simulink model "PubIfDecisionTOS_MDL"  (R2020b)
settings: configuration reference "DspaceConfig" (kept outside this file)
PostLoadFcn:
  | if any(exist('dsrtsu_mdlpostloadfcn', 'file') ~= 0), dsrtsu_mdlpostloadfcn('Execute', bdroot); end
InitFcn:
  | , if any(exist('dsmpb_private', 'file') ~= 0), dsmpb_private('dsmpb_mdlclblib', 'Init', bdroot); end,
undefined symbols (not defined in the file or in its folder): C_TOS_ACCEgoRAxletoFbumplength_m, C_TOS_ACCTargetFront_Flag, C_TOS_AEBJAPedObjDxThre_Val, C_TOS_AEBJAPedObjDyThre_Val, C_TOS_AEBJATargetSize_Val, C_TOS_AEBJAVehObjDxThre_Val, C_TOS_AEBJAVehObjDyThre_Val, C_TOS_AEBJuncPedTargetSize_Val, C_TOS_AEBLatObjDxThre_Val, C_TOS_AEBLatPedDyThre_Val, C_TOS_AEBLatTargetSize_Val, C_TOS_AEBLongTargetInEgoFront_Flag, C_TOS_axAbsGround_Parameter, C_TOS_CameraConfirmedFlag, C_TOS_CNsubjWidth, C_TOS_CurrentLaneCoreMinWidth_Val, C_TOS_CutInProb_Val_Zero, C_TOS_CutOutProb_Val_Zero, C_TOS_D2R_Val, C_TOS_DefaultValueObjectToCenterLine_dy, C_TOS_EgoCarWidth_Val, C_TOS_EgoDxRefPoint_m, C_TOS_EgoRAxletoFbumplength_m, C_TOS_HalfWidthVehicle_Con, C_TOS_HWA_CurrentLaneFlag, C_TOS_HWA_LeftLaneFlag, C_TOS_HWA_MovingDir_Vaild, C_TOS_HWA_MovState_Vaild, C_TOS_HWA_RightLaneFlag, C_TOS_LaneLineCourseErrorFront, C_TOS_LaneLineCourseErrorRear, C_TOS_MotorbikeDefaultWidth_m, C_TOS_NumberOfEffectiveTargets, C_TOS_Obj_Age_Val, C_TOS_Objdx_Constraint_Val, C_TOS_ObjectDefaultWidth_m, C_TOS_ObjInCurrentLane_Val, C_TOS_ObjInCurrentLaneValid, C_TOS_ObjInLeftLaneValid, C_TOS_ObjInRightLaneValid, C_TOS_ObjNotInCurrentLane_Val, C_TOS_ObjNotREElementType, C_TOS_ObjPredictDis_dy_ConstantVal_Zeros, C_TOS_ObjToCenterLine_ConstantVal_Zeros, C_TOS_OFMObjIDInvilad_Val, C_TOS_PIL_LatDisCons_Val_zero, C_TOS_PIL_ObjectCutInFlag_b, C_TOS_PIL_ObjectCutOutFlag_b, C_TOS_PIL_ObjLaneProb_al_Val, C_TOS_PP_ObjFusType_FC_Confirm_b, C_TOS_PP_ObjFusType_FC_FR_Confirm_b, C_TOS_PP_ObjFusType_FR_Confirm_b, C_TOS_RE_80BoolDefault_Val, C_TOS_RE_80Single181Default_Val, C_TOS_RE_80Single255Default_Val, C_TOS_RE_80Uint8Default_Val, C_TOS_RE_D2R, C_TOS_RE_D_180_Val, C_TOS_RE_InvalidObjectID_Val, C_TOS_RE_InvalidTargetChainDir_Val ... (+142)
libraries: simulink x1650, TOS_LIB x361, canfdmsglib x14
(part 7 of 69)

== system PubIfDecisionTOS_MDL/TOS_20201112/TOS_2012080320/TOS/ACC/TOS_ACCCurrentLane ==
  TOSAAt_OFM_TIL_VIE : Inport
  ACCTargetInfor : Subsystem
  ACC_CurrentLane_Target : Subsystem
  ACC_Object_PreConfirm : Subsystem
  Bus Selector : BusSelector  OutputSignals=IDP0,dxP0
  Bus Selector1 : BusSelector  OutputSignals=VIE_SignalVerification.vxvRefMs,OFM_SignalVerification,TOS_AddAttributes,TLJ_TargetInLaneValidityJudg.TOS_TLJ_SameLaneConfirm_Flag,TOS_ProbInLaneCalculat,TOS_VCAN_SignalVerification,LM_SignalVerification.TOS_LM_LR_Bus.LM_LR_Line04.dDisStart,LM_SignalVerification.TOS_LM_LR_Bus.LM_LR_Line04.dDisEnd,LM_SignalVerification.TOS_LM_LR_Bus.LM_LR_Line05.dDisStart,LM_SignalVerification.TOS_LM_LR_Bus.LM_LR_Line05.dDisEnd,LM_SignalVerification.TOS_LM_LR_Bus.LM_LR_Line06.dDisStart,LM_SignalVerification.TOS_LM_LR_Bus.LM_LR_Line06.dDisEnd,LM_SignalVerification.TOS_LM_LR_Bus.LM_LR_Line04.pC2,LM_SignalVerification.TOS_LM_LR_Bus.LM_LR_Line05.pC2,LM_SignalVerification.TOS_LM_LR_Bus.LM_LR_Line06.pC2,LM_SignalVerification.TOS_LM_LR_Bus.LM_LR_Line04.fCamValid,LM_SignalVerification.TOS_LM_LR_Bus.LM_LR_Line05.fCamValid,LM_SignalVerification.TOS_LM_LR_Bus.LM_LR_Line06.fCamValid,LM_SignalVerification.TOS_LM_LR_Bus.LM_LR_Line04.pC0,LM_SignalVerification.TOS_LM_RL_Bus.LM_RL_Line04.pC0,LM_SignalVerification.TOS_LM_LR_Bus.LM_LR_Line04.pC1,LM_SignalVerification.TOS_LM_RL_Bus.LM_RL_Line04.pC1
  Bus Selector2 : BusSelector  OutputSignals=OFM_SignalVerification,TOS_AddAttributes,TOS_ProbInLaneCalculat
  Bus Selector3 : BusSelector  OutputSignals=IDP0,ObjMovingStateP0
  Bus Selector4 : BusSelector  OutputSignals=OFM_SignalVerification.Object_DX,OFM_SignalVerification.Object_ID
  Bus Selector5 : BusSelector  OutputSignals=TOS_AddAttributes.PP_ObjFusType_FC_FR_Confirm,TOS_AddAttributes.PP_ObjFusType_FR_Confirm,TOS_AddAttributes.PP_ObjFusType_FC_Confirm,OFM_SignalVerification.Object_ID,OFM_SignalVerification.Object_MovingState,OFM_SignalVerification.Object_DX,OFM_SignalVerification.Object_ObstacleProb,OFM_SignalVerification.Object_DY,OFM_SignalVerification.Object_Type,TLJ_TargetInLaneValidityJudg.TOS_TLJ_SameLaneConfirm_Flag,LM_SignalVerification.TOS_LM_LR_Bus.LM_LR_Line04.fCamValid,LM_SignalVerification.TOS_LM_LR_Bus.LM_LR_Line05.fCamValid,LM_SignalVerification.TOS_LM_LR_Bus.LM_LR_Line06.fCamValid,TOS_ProbInLaneCalculat.PIL_OverlapRatio,LM_SignalVerification.TOS_LM_LR_Bus.LM_LR_Line04.dDisStart,LM_SignalVerification.TOS_LM_LR_Bus.LM_LR_Line04.dDisEnd,LM_SignalVerification.TOS_LM_LR_Bus.LM_LR_Line05.dDisStart,LM_SignalVerification.TOS_LM_LR_Bus.LM_LR_Line05.dDisEnd,LM_SignalVerification.TOS_LM_LR_Bus.LM_LR_Line06.dDisStart,LM_SignalVerification.TOS_LM_LR_Bus.LM_LR_Line06.dDisEnd,PP_REElementType
  Bus Selector6 : BusSelector  OutputSignals=IDP1,ObjMovingStateP1
  Bus Selector7 : BusSelector  OutputSignals=TOS_ACC_P0_P1_TargetPre_SameLaneFlag,TOS_ACC_P0_P1_TargetPreFiltFlag
  Constant1 : Constant  Value=C_TOS_NumberOfEffectiveTargets  OutDataTypeStr=uint8
      settings: AttributesFormatString=C_TOS_NumberOfEffectiveTargets = 80
  MATLAB Function1 : MATLAB Function  TreatAsAtomicUnit=on
  Terminator1 : Terminator
  Terminator2 : Terminator
  Vector Concatenate : Concatenate
  TOS_ACCP0 : Outport  PortDimensions=1  BusOutputAsStruct=on
  TOS_ACCP1 : Outport  Port=2
  wires:
  ACCTargetInfor/2(TOS_ACCP1) -> TOS_ACCP1/1, [TOS_ACCP1]
  Bus Selector2/2 -> ACCTargetInfor/2(TOS_AddAttributes)  "<TOS_AddAttributes>"
  Bus Selector2/1 -> ACCTargetInfor/1(OFM_SignalVerification)  "<OFM_SignalVerification>"
  Bus Selector2/3 -> ACCTargetInfor/3(TOS_ProbInLaneCalculat)  "<TOS_ProbInLaneCalculat>"
  Bus Selector1/1 -> ACC_CurrentLane_Target/1(VIE_EgoVelocity)  "<vxvRefMs>"
  Bus Selector1/2 -> ACC_CurrentLane_Target/2(OFM_SignalVerification)  "<OFM_SignalVerification>"
  Bus Selector1/3 -> ACC_CurrentLane_Target/3(TOS_AddAttributes)  "<TOS_AddAttributes>"
  Bus Selector1/4 -> ACC_CurrentLane_Target/4(TOS_TLJ_SameLaneConfirm_Flag)  "<TOS_TLJ_SameLaneConfirm_Flag>"
  Bus Selector1/5 -> ACC_CurrentLane_Target/5(TOS_ProbInLaneCalculat)  "<TOS_ProbInLaneCalculat>"
  MATLAB Function1/2(Dx2edNearestObjIndex) -> Vector Concatenate/2
  MATLAB Function1/1(Dx1stNearestObjIndex) -> Vector Concatenate/1
  Bus Selector4/1 -> MATLAB Function1/1(Object_Dx)  "<Object_DX>"
  Bus Selector4/2 -> MATLAB Function1/2(Object_ID)  "<Object_ID>"
  Constant1/1 -> MATLAB Function1/5(Object_Num)
  Bus Selector1/6 -> ACC_CurrentLane_Target/6(TOS_VCAN_SignalVerification)  "<TOS_VCAN_SignalVerification>"
  ACCTargetInfor/1(TOS_ACCP0) -> [TOS_ACCP0], TOS_ACCP0/1
  [TOS_ACCP0] -> Bus Selector/1
  Bus Selector/1 -> ACC_Object_PreConfirm/22(ACC_TargetP0_ID_K1)  "<IDP0>"
  Bus Selector/2 -> ACC_Object_PreConfirm/23(ACC_TargetP0_Dx_K1)  "<dxP0>"
  TOSAAt_OFM_TIL_VIE/1 -> Bus Selector5/1, Bus Selector1/1, Bus Selector2/1, Bus Selector4/1
  Vector Concatenate/1 -> ACC_CurrentLane_Target/23(ACC_P0_P1_Index)  "TOS_ACC_P0_P1_Index"
  ACC_CurrentLane_Target/1(TOS_ACC_P0_TragetIndex) -> ACCTargetInfor/4(TOS_ACCP0TargetIndex)
  ACC_CurrentLane_Target/2(TOS_ACC_P1_TragetIndex) -> ACCTargetInfor/5(TOS_ACCP1TargetIndex)
  [TOS_ACCP0] -> Bus Selector3/1
  Bus Selector3/1 -> ACC_CurrentLane_Target/24(ACC_TargetP0_ID_K1)  "<IDP0>"
  Bus Selector3/2 -> ACC_CurrentLane_Target/25(ACC_TargetP0_MovState_K1)  "<ObjMovingStateP0>"
  [TOS_ACCP1] -> Bus Selector6/1
  Bus Selector6/1 -> ACC_CurrentLane_Target/26(ACC_TargetP1_ID_K1)  "<IDP1>"
  Bus Selector6/2 -> ACC_CurrentLane_Target/27(ACC_TargetP1_MovState_K1)  "<ObjMovingStateP1>"
  ACC_Object_PreConfirm/1(TOS_ACC_P0_P1_TargetPreConfirm) -> Bus Selector7/1
  Bus Selector7/1 -> MATLAB Function1/3(ConditionJudge)  "<TOS_ACC_P0_P1_TargetPre_SameLaneFlag>"
  Bus Selector7/2 -> MATLAB Function1/4(TargetFusionTypeFlag)  "<TOS_ACC_P0_P1_TargetPreFiltFlag>"
  MATLAB Function1/3(Dx1stNearestObjID) -> Terminator1/1
  MATLAB Function1/4(Dx2edNearestObjID) -> Terminator2/1
  Bus Selector1/7 -> ACC_CurrentLane_Target/7(LM_LR_Line04_dDisStart)  "<dDisStart>"
  Bus Selector1/8 -> ACC_CurrentLane_Target/8(LM_LR_Line04_dDisEnd)  "<dDisEnd>"
  Bus Selector1/9 -> ACC_CurrentLane_Target/9(LM_LR_Line05_dDisStart)  "<dDisStart>"
  Bus Selector1/10 -> ACC_CurrentLane_Target/10(LM_LR_Line05_dDisEnd)  "<dDisEnd>"
  Bus Selector1/11 -> ACC_CurrentLane_Target/11(LM_LR_Line06_dDisStart)  "<dDisStart>"
  Bus Selector1/12 -> ACC_CurrentLane_Target/12(LM_LR_Line06_dDisEnd)  "<dDisEnd>"
  Bus Selector1/13 -> ACC_CurrentLane_Target/13(LM_LR_Line04_pC2)  "<pC2>"
  Bus Selector1/14 -> ACC_CurrentLane_Target/14(LM_LR_Line05_pC2)  "<pC2>"
  Bus Selector1/15 -> ACC_CurrentLane_Target/15(LM_LR_Line06_pC2)  "<pC2>"
  Bus Selector1/16 -> ACC_CurrentLane_Target/16(LM_LR_Line04_fCamValid)  "<fCamValid>"
  Bus Selector1/17 -> ACC_CurrentLane_Target/17(LM_LR_Line05_fCamValid)  "<fCamValid>"
  Bus Selector1/18 -> ACC_CurrentLane_Target/18(LM_LR_Line06_fCamValid)  "<fCamValid>"
  Bus Selector1/19 -> ACC_CurrentLane_Target/19(LM_LR_Line04_pC0)  "<pC0>"
  Bus Selector1/20 -> ACC_CurrentLane_Target/20(LM_RL_Line04_pC0)  "<pC0>"
  Bus Selector1/21 -> ACC_CurrentLane_Target/21(LM_LR_Line04_pC1)  "<pC1>"
  Bus Selector1/22 -> ACC_CurrentLane_Target/22(LM_RL_Line04_pC1)  "<pC1>"
  Bus Selector5/12 -> ACC_Object_PreConfirm/12(LM_LR_Line05_fCamValid)  "<fCamValid>"
  Bus Selector5/11 -> ACC_Object_PreConfirm/11(LM_LR_Line04_fCamValid)  "<fCamValid>"
  Bus Selector5/13 -> ACC_Object_PreConfirm/13(LM_LR_Line06_fCamValid)  "<fCamValid>"
  Bus Selector5/21 -> ACC_Object_PreConfirm/21(PP_REElementType)  "<PP_REElementType>"
  Bus Selector5/10 -> ACC_Object_PreConfirm/10(TOS_TLJ_SameLaneConfirm_Flag)  "<TOS_TLJ_SameLaneConfirm_Flag>"
  Bus Selector5/14 -> ACC_Object_PreConfirm/14(PIL_OverlapRatio)  "<PIL_OverlapRatio>"
  Bus Selector5/9 -> ACC_Object_PreConfirm/9(Object_Type)  "<Object_Type>"
  Bus Selector5/15 -> ACC_Object_PreConfirm/15(LM_LR_Line04_dDisStart)  "<dDisStart>"
  Bus Selector5/8 -> ACC_Object_PreConfirm/8(Object_DY)  "<Object_DY>"
  Bus Selector5/16 -> ACC_Object_PreConfirm/16(LM_LR_Line04_dDisEnd)  "<dDisEnd>"
  Bus Selector5/7 -> ACC_Object_PreConfirm/7(Object_ObstacleProb)  "<Object_ObstacleProb>"
  Bus Selector5/17 -> ACC_Object_PreConfirm/17(LM_LR_Line05_dDisStart)  "<dDisStart>"
  Bus Selector5/6 -> ACC_Object_PreConfirm/6(Obj_Dx)  "<Object_DX>"
  Bus Selector5/18 -> ACC_Object_PreConfirm/18(LM_LR_Line05_dDisEnd)  "<dDisEnd>"
  Bus Selector5/5 -> ACC_Object_PreConfirm/5(Obj_MovingState)  "<Object_MovingState>"
  Bus Selector5/19 -> ACC_Object_PreConfirm/19(LM_LR_Line06_dDisStart)  "<dDisStart>"
  Bus Selector5/4 -> ACC_Object_PreConfirm/4(Object_ID)  "<Object_ID>"
  Bus Selector5/20 -> ACC_Object_PreConfirm/20(LM_LR_Line06_dDisEnd)  "<dDisEnd>"
  Bus Selector5/3 -> ACC_Object_PreConfirm/3(PP_ObjFusType_FC_Confirm)  "<PP_ObjFusType_FC_Confirm>"
  Bus Selector5/2 -> ACC_Object_PreConfirm/2(PP_ObjFusType_FR_Confirm)  "<PP_ObjFusType_FR_Confirm>"
  Bus Selector5/1 -> ACC_Object_PreConfirm/1(PP_ObjFusType_FC_FR_Confirm)  "<PP_ObjFusType_FC_FR_Confirm>"

== system PubIfDecisionTOS_MDL/TOS_20201112/TOS_2012080320/TOS/ACC/TOS_ACCLeftLane ==
  TOSAAt_OFM_TIL_VIE : Inport
  ACCTargetPO24Infor : Subsystem
  ACC_LeftLane_Target : Subsystem
  ACC_Object_PreConfirm : Subsystem
  Bus Selector : BusSelector  OutputSignals=IDP2,dxP2
  Bus Selector1 : BusSelector  OutputSignals=VIE_SignalVerification.vxvRefMs,OFM_SignalVerification,TOS_AddAttributes,TOS_ProbInLaneCalculat,TOS_VCAN_SignalVerification
  Bus Selector2 : BusSelector  OutputSignals=OFM_SignalVerification,TOS_AddAttributes,TOS_ProbInLaneCalculat
  Bus Selector3 : BusSelector  OutputSignals=TOS_ACC_P2_P4_TargetPre_Confirm_FiltFlag
  Bus Selector4 : BusSelector  OutputSignals=OFM_SignalVerification.Object_DX,OFM_SignalVerification.Object_ID,TLJ_TargetInLaneValidityJudg.TOS_TLJ_LeftLaneConfirm_Flag
  Bus Selector5 : BusSelector  OutputSignals=TOS_AddAttributes.PP_ObjFusType_FC_FR_Confirm,TOS_AddAttributes.PP_ObjFusType_FR_Confirm,TOS_AddAttributes.PP_ObjFusType_FC_Confirm,OFM_SignalVerification.Object_ID,OFM_SignalVerification.Object_MovingState,OFM_SignalVerification.Object_DX,OFM_SignalVerification.Object_ObstacleProb,OFM_SignalVerification.Object_DY,OFM_SignalVerification.Object_Type
  Bus Selector6 : BusSelector  OutputSignals=IDP2,ObjMovingStateP2
  Constant1 : Constant  Value=C_TOS_NumberOfEffectiveTargets  OutDataTypeStr=uint8
      settings: AttributesFormatString=C_TOS_NumberOfEffectiveTargets = 80
  MATLAB Function1 : MATLAB Function  TreatAsAtomicUnit=on
  Terminator : Terminator
  Terminator2 : Terminator
  Vector Concatenate : Concatenate
  TOS_ACCPO2 : Outport  PortDimensions=1  BusOutputAsStruct=on
  TOS_ACCPO4 : Outport  Port=2
  wires:
  Bus Selector1/4 -> ACC_LeftLane_Target/4(TOS_ProbInLaneCalculat)  "<TOS_ProbInLaneCalculat>"
  Bus Selector2/2 -> ACCTargetPO24Infor/2(TOS_AddAttributes)  "<TOS_AddAttributes>"
  Bus Selector2/1 -> ACCTargetPO24Infor/1(OFM_SignalVerification)  "<OFM_SignalVerification>"
  Bus Selector2/3 -> ACCTargetPO24Infor/3(TOS_ProbInLaneCalculat)  "<TOS_ProbInLaneCalculat>"
  Bus Selector1/1 -> ACC_LeftLane_Target/1(VIE_EgoVelocity)  "<vxvRefMs>"
  Bus Selector1/2 -> ACC_LeftLane_Target/2(OFM_SignalVerification)  "<OFM_SignalVerification>"
  Bus Selector1/3 -> ACC_LeftLane_Target/3(TOS_AddAttributes)  "<TOS_AddAttributes>"
  ACCTargetPO24Infor/1(TOS_ACCPO2) -> [TOS_ACCP2], TOS_ACCPO2/1
  ACCTargetPO24Infor/2(TOS_ACCPO4) -> TOS_ACCPO4/1
  Vector Concatenate/1 -> ACC_LeftLane_Target/6(TOS_ACC_P2_P4_Index)  "TOS_ACC_P2_P4_Index"
  MATLAB Function1/3(Dx1stNearestObjID) -> Terminator/1
  Bus Selector4/1 -> MATLAB Function1/1(Object_Dx)  "<Object_DX>"
  Bus Selector4/3 -> MATLAB Function1/3(ConditionJudge)  "<TOS_TLJ_LeftLaneConfirm_Flag>"
  Bus Selector4/2 -> MATLAB Function1/2(Object_ID)  "<Object_ID>"
  MATLAB Function1/1(Dx1stNearestObjIndex) -> Vector Concatenate/1
  MATLAB Function1/2(Dx2edNearestObjIndex) -> Vector Concatenate/2
  MATLAB Function1/4(Dx2edNearestObjID) -> Terminator2/1
  ACC_LeftLane_Target/1(TOS_ACC_P2_TragetIndex) -> ACCTargetPO24Infor/4(TOS_ACCPO2TargetIndex)
  Constant1/1 -> MATLAB Function1/5(Object_Num)
  Bus Selector3/1 -> MATLAB Function1/4(TOS_ACC_P2_P4_TargetPre_Confirm_FiltFlag)  "<TOS_ACC_P2_P4_TargetPre_Confirm_FiltFlag>"
  Bus Selector/2 -> ACC_Object_PreConfirm/11(ACC_Target_Dx_K1)  "<dxP2>"
  TOSAAt_OFM_TIL_VIE/1 -> Bus Selector1/1, Bus Selector2/1, Bus Selector4/1, Bus Selector5/1
  Bus Selector/1 -> ACC_Object_PreConfirm/10(ACC_Target_ID_K1)  "<IDP2>"
  [TOS_ACCP2] -> Bus Selector/1
  Bus Selector5/7 -> ACC_Object_PreConfirm/7(Object_ObstacleProb)  "<Object_ObstacleProb>"
  Bus Selector5/9 -> ACC_Object_PreConfirm/9(Object_Type)  "<Object_Type>"
  Bus Selector5/6 -> ACC_Object_PreConfirm/6(Obj_Dx)  "<Object_DX>"
  Bus Selector5/8 -> ACC_Object_PreConfirm/8(Object_DY)  "<Object_DY>"
  Bus Selector5/5 -> ACC_Object_PreConfirm/5(Obj_MovingState)  "<Object_MovingState>"
  Bus Selector5/4 -> ACC_Object_PreConfirm/4(Object_ID)  "<Object_ID>"
  Bus Selector5/3 -> ACC_Object_PreConfirm/3(PP_ObjFusType_FC_Confirm)  "<PP_ObjFusType_FC_Confirm>"
  Bus Selector5/2 -> ACC_Object_PreConfirm/2(PP_ObjFusType_FR_Confirm)  "<PP_ObjFusType_FR_Confirm>"
  Bus Selector5/1 -> ACC_Object_PreConfirm/1(PP_ObjFusType_FC_FR_Confirm)  "<PP_ObjFusType_FC_FR_Confirm>"
  ACC_Object_PreConfirm/1(TOS_ACC_P2_P4_TargetPreConfirm) -> Bus Selector3/1
  Bus Selector1/5 -> ACC_LeftLane_Target/5(TOS_VCAN_SignalVerification)  "<TOS_VCAN_SignalVerification>"
  Bus Selector6/1 -> ACC_LeftLane_Target/7(ACC_TargetP2_ID_K1)  "<IDP2>"
  Bus Selector6/2 -> ACC_LeftLane_Target/8(ACC_TargetP2_MovState_K1)  "<ObjMovingStateP2>"
  [TOS_ACCP2] -> Bus Selector6/1
  ACC_LeftLane_Target/2(TOS_ACC_P4_TragetIndex) -> [TOS_ACCP4], ACCTargetPO24Infor/5(TOS_ACCPO4TargetIndex)
  [TOS_ACCP4] -> ACC_LeftLane_Target/9(ACC_TargetP4_ID_K1)

== system PubIfDecisionTOS_MDL/TOS_20201112/TOS_2012080320/TOS/ACC/TOS_ACCRightLane ==
  TOSAAt_OFM_TIL_VIE : Inport
  ACCTargetPO35Infor : Subsystem
  ACC_LeftLane_Target : Subsystem
  ACC_Object_PreConfirm : Subsystem
  Bus Selector : BusSelector  OutputSignals=IDP3,dxP3
  Bus Selector1 : BusSelector  OutputSignals=VIE_SignalVerification.vxvRefMs,OFM_SignalVerification,TOS_AddAttributes,TOS_ProbInLaneCalculat,TOS_VCAN_SignalVerification
  Bus Selector2 : BusSelector  OutputSignals=OFM_SignalVerification,TOS_AddAttributes,TOS_ProbInLaneCalculat
  Bus Selector3 : BusSelector  OutputSignals=TOS_ACC_P3_P5_TargetPre_Confirm_FiltFlag
  Bus Selector4 : BusSelector  OutputSignals=OFM_SignalVerification.Object_DX,OFM_SignalVerification.Object_ID,TLJ_TargetInLaneValidityJudg.TOS_TLJ_RightLaneConfirm_Flag
  Bus Selector5 : BusSelector  OutputSignals=TOS_AddAttributes.PP_ObjFusType_FC_FR_Confirm,TOS_AddAttributes.PP_ObjFusType_FR_Confirm,TOS_AddAttributes.PP_ObjFusType_FC_Confirm,OFM_SignalVerification.Object_ID,OFM_SignalVerification.Object_MovingState,OFM_SignalVerification.Object_DX,OFM_SignalVerification.Object_ObstacleProb,OFM_SignalVerification.Object_DY,OFM_SignalVerification.Object_Type
  Bus Selector6 : BusSelector  OutputSignals=IDP3,ObjMovingStateP3
  Constant1 : Constant  Value=C_TOS_NumberOfEffectiveTargets  OutDataTypeStr=uint8
      settings: AttributesFormatString=C_TOS_NumberOfEffectiveTargets = 80
  MATLAB Function1 : MATLAB Function  TreatAsAtomicUnit=on
  Terminator : Terminator
  Terminator2 : Terminator
  Vector Concatenate : Concatenate
  TOS_ACCP3 : Outport  PortDimensions=1  BusOutputAsStruct=on
  TOS_ACCP5 : Outport  Port=2
  wires:
  ACCTargetPO35Infor/1(TOS_ACCPO3) -> [TOS_ACCP3], TOS_ACCP3/1
  ACCTargetPO35Infor/2(TOS_ACCPO5) -> TOS_ACCP5/1
  Bus Selector2/2 -> ACCTargetPO35Infor/2(TOS_AddAttributes)  "<TOS_AddAttributes>"
  Bus Selector2/1 -> ACCTargetPO35Infor/1(OFM_SignalVerification)  "<OFM_SignalVerification>"
  Bus Selector2/3 -> ACCTargetPO35Infor/3(TOS_ProbInLaneCalculat)  "<TOS_ProbInLaneCalculat>"
  MATLAB Function1/3(Dx1stNearestObjID) -> Terminator/1
  MATLAB Function1/4(Dx2edNearestObjID) -> Terminator2/1
  Bus Selector4/1 -> MATLAB Function1/1(Object_Dx)  "<Object_DX>"
  MATLAB Function1/2(Dx2edNearestObjIndex) -> Vector Concatenate/2
  Vector Concatenate/1 -> ACC_LeftLane_Target/6(TOS_ACC_P3_P5_Index)  "TOS_ACC_P3_P5_Index"
  MATLAB Function1/1(Dx1stNearestObjIndex) -> Vector Concatenate/1
  Bus Selector4/2 -> MATLAB Function1/2(Object_ID)  "<Object_ID>"
  Bus Selector4/3 -> MATLAB Function1/3(ConditionJudge)  "<TOS_TLJ_RightLaneConfirm_Flag>"
  ACC_LeftLane_Target/1(TOS_ACC_P3_TragetIndex) -> ACCTargetPO35Infor/4(TOS_ACCPO3TargetIndex)
  ACC_LeftLane_Target/2(TOS_ACC_P5_TragetIndex) -> [TOS_ACCP5], ACCTargetPO35Infor/5(TOS_ACCPO5TargetIndex)
  ACC_Object_PreConfirm/1(TOS_ACC_P3_P5_TargetPreConfirm) -> Bus Selector3/1
  Bus Selector5/1 -> ACC_Object_PreConfirm/1(PP_ObjFusType_FC_FR_Confirm)  "<PP_ObjFusType_FC_FR_Confirm>"
  Bus Selector5/2 -> ACC_Object_PreConfirm/2(PP_ObjFusType_FR_Confirm)  "<PP_ObjFusType_FR_Confirm>"
  Bus Selector5/3 -> ACC_Object_PreConfirm/3(PP_ObjFusType_FC_Confirm)  "<PP_ObjFusType_FC_Confirm>"
  Bus Selector5/4 -> ACC_Object_PreConfirm/4(Object_ID)  "<Object_ID>"
  Bus Selector5/5 -> ACC_Object_PreConfirm/5(Obj_MovingState)  "<Object_MovingState>"
  Bus Selector5/8 -> ACC_Object_PreConfirm/8(Object_DY)  "<Object_DY>"
  Bus Selector5/6 -> ACC_Object_PreConfirm/6(Obj_Dx)  "<Object_DX>"
  Bus Selector5/9 -> ACC_Object_PreConfirm/9(Object_Type)  "<Object_Type>"
  Bus Selector5/7 -> ACC_Object_PreConfirm/7(Object_ObstacleProb)  "<Object_ObstacleProb>"
  [TOS_ACCP3] -> Bus Selector/1
  Bus Selector/1 -> ACC_Object_PreConfirm/10(ACC_Target_ID_K1)  "<IDP3>"
  Bus Selector/2 -> ACC_Object_PreConfirm/11(ACC_Target_Dx_K1)  "<dxP3>"
  Bus Selector3/1 -> MATLAB Function1/4(TargetFusionTypeFlag)  "<TOS_ACC_P3_P5_TargetPre_Confirm_FiltFlag>"
  Constant1/1 -> MATLAB Function1/5(Object_Num)
  [TOS_ACCP3] -> Bus Selector6/1
  Bus Selector6/2 -> ACC_LeftLane_Target/8(ACC_TargetP3_MovState_K1)  "<ObjMovingStateP3>"
  Bus Selector1/3 -> ACC_LeftLane_Target/3(TOS_AddAttributes)  "<TOS_AddAttributes>"
  Bus Selector1/2 -> ACC_LeftLane_Target/2(OFM_SignalVerification)  "<OFM_SignalVerification>"
  Bus Selector1/1 -> ACC_LeftLane_Target/1(VIE_EgoVelocity)  "<vxvRefMs>"
  TOSAAt_OFM_TIL_VIE/1 -> Bus Selector5/1, Bus Selector1/1, Bus Selector2/1, Bus Selector4/1
  Bus Selector1/4 -> ACC_LeftLane_Target/4(TOS_ProbInLaneCalculat)  "<TOS_ProbInLaneCalculat>"
  Bus Selector1/5 -> ACC_LeftLane_Target/5(TOS_VCAN_SignalVerification)  "<TOS_VCAN_SignalVerification>"
  Bus Selector6/1 -> ACC_LeftLane_Target/7(ACC_TargetP3_ID_K1)  "<IDP3>"
  [TOS_ACCP5] -> ACC_LeftLane_Target/9(ACC_TargetP5_ID_K1)

== system PubIfDecisionTOS_MDL/TOS_20201112/TOS_2012080320/TOS/AEB/TOS_AEBJunct1105 ==
  TOSAAt_OFM_TIL_VIE : Inport
  AEBJuncTargetIndex : Subsystem
  AEBJunc_Object_Condition : Subsystem
  AEBJunc_Object_Condition1 : Subsystem  Commented=on
  AEBJunctionTargetInfor : Subsystem
  Bus Creator : BusCreator  Inputs=9
  Bus Selector1 : BusSelector  Commented=on  OutputSignals=OFM_SignalVerification.Object_ID,TOS_AddAttributes.PP_ObjFusType_FC_FR_Confirm,TOS_AddAttributes.PP_ObjFusType_FR_Confirm,OFM_SignalVerification.Object_Type,OFM_SignalVerification.Object_DX,OFM_SignalVerification.Object_DY,TOS_AddAttributes.PP_ObjMovingDirSignalProcessing,OFM_SignalVerification.Object_HeadingAngle,OFM_SignalVerification.Object_VX,OFM_SignalVerification.Object_VY,VIE_SignalVerification.vxvRefMs,VIE_SignalVerification.psiDtOpt,VIE_SignalVerification.axvRefMs2,OFM_SignalVerification.Object_MovingState
  Bus Selector2 : BusSelector  OutputSignals=OFM_SignalVerification,TOS_AddAttributes
  Bus Selector3 : BusSelector  OutputSignals=OFM_SignalVerification.Object_ID,TOS_AddAttributes.PP_ObjFusType_FC_FR_Confirm,TOS_AddAttributes.PP_ObjFusType_FR_Confirm,OFM_SignalVerification.Object_Type,OFM_SignalVerification.Object_DX,OFM_SignalVerification.Object_DY,TOS_AddAttributes.PP_ObjMovingDirSignalProcessing,OFM_SignalVerification.Object_HeadingAngle,OFM_SignalVerification.Object_VX,OFM_SignalVerification.Object_VY,VIE_SignalVerification.vxvRefMs,VIE_SignalVerification.psiDtOpt,VIE_SignalVerification.axvRefMs2,OFM_SignalVerification.Object_MovingState
  Display{,1..10} (11 alike) : Display  Commented=on
  From2 : From  Commented=on  GotoTag=TOS_AEB_JAOBJ
  From3 : From  Commented=on  GotoTag=TOS_AEBJunc_TargetIndex
  From4 : From  Commented=on  GotoTag=TOS_AEBJunc_ObserVale
  Selector{1..10,14} (11 alike) : Selector  Commented=on  InputPortWidth=80  IndexOptions=Index vector (dialog)  Indices=60  OutputSizes=1
  Subsystem : Subsystem
  Subsystem1 : Subsystem
  Subsystem2 : Subsystem  Commented=on
  TOS_AEBLong_ObserVale : Subsystem  Commented=on
  Unit Delay{,1..3} (4 alike) : UnitDelay  SampleTime=-1  HasFrameUpgradeWarning=on
  Unit Delay4 : UnitDelay  Commented=on  SampleTime=-1  HasFrameUpgradeWarning=on
  Unit Delay5 : UnitDelay  Commented=on  SampleTime=-1  HasFrameUpgradeWarning=on
  TOS_AEB_JAOBJ : Outport
  wires:
  AEBJuncTargetIndex/1(TOS_AEBJuncTargetIndex) -> [TOS_AEBJunc_TargetIndex], AEBJunctionTargetInfor/3(TOS_AEBJuncTargetIndex)  "TOS_AEBJunc_Index"
  AEBJunc_Object_Condition/1(TOS_AEBJunc_PedTargets_Dx) -> AEBJuncTargetIndex/1(TOS_AEBJunc_ConditionPedTargets_Dx)  "TOS_AEBJunc_ConditionPedTargets_Dx"
  AEBJunctionTargetInfor/1(TOS_AEB_JAOBJ) -> [TOS_AEB_JAOBJ], TOS_AEB_JAOBJ/1
  Bus Selector2/1 -> AEBJunctionTargetInfor/1(OFM_SignalVerification)  "<OFM_SignalVerification>"
  Bus Selector2/2 -> AEBJunctionTargetInfor/2(TOS_AddAttributes)  "<TOS_AddAttributes>"
  Bus Selector3/5 -> AEBJunc_Object_Condition/5(Object_Dx)  "<Object_DX>"
  Bus Selector3/7 -> AEBJunc_Object_Condition/7(PP_ObjMovingDirSignalProcessing)  "<PP_ObjMovingDirSignalProcessing>"
  Subsystem/1(ObjectID) -> Unit Delay/1
  [TOS_AEB_JAOBJ] -> Subsystem/1(TOS_AEB_JAOBJ)
  Bus Selector3/6 -> AEBJunc_Object_Condition/6(Object_Dy)  "<Object_DY>"
  Bus Selector3/4 -> AEBJunc_Object_Condition/4(ObjectType)  "<Object_Type>"
  Bus Selector3/10 -> AEBJunc_Object_Condition/10(Object_VY)  "<Object_VY>"
  Bus Selector3/8 -> AEBJunc_Object_Condition/8(Object_HeadingAngle)  "<Object_HeadingAngle>"
  Bus Selector3/2 -> AEBJunc_Object_Condition/2(PP_ObjFusType_FC_FR_Confirm)  "<PP_ObjFusType_FC_FR_Confirm>"
  Unit Delay/1 -> AEBJunc_Object_Condition/15(AEBJunc_Target_ObjectID_K1)
  Bus Selector3/9 -> AEBJunc_Object_Condition/9(Object_VX)  "<Object_VX>"
  Bus Selector3/1 -> AEBJunc_Object_Condition/1(Object_ID)  "<Object_ID>"
  Bus Selector3/11 -> AEBJunc_Object_Condition/11(VIE_EgoVelocity)  "<vxvRefMs>"
  Bus Selector3/3 -> AEBJunc_Object_Condition/3(PP_ObjFusType_FR_Confirm)  "<PP_ObjFusType_FR_Confirm>"
  Bus Selector3/12 -> AEBJunc_Object_Condition/12(psiDtOpt)  "<psiDtOpt>"
  Bus Selector3/13 -> AEBJunc_Object_Condition/13(axvRefMs2)  "<axvRefMs2>"
  AEBJunc_Object_Condition/3(AEBJunc_PedTargetFusionType_observal) -> Bus Creator/1  "AEBJunc_PedTargetFusionType_observal"
  Subsystem/2(ObjectType) -> Unit Delay1/1
  Unit Delay1/1 -> AEBJunc_Object_Condition/16(AEBJunc_Target_ObjectType_K1)
  AEBJunc_Object_Condition/4(AEBJunc_PedTargetObjectType_observal) -> Bus Creator/2  "AEBJunc_PedTargetObjectType_observal"
  AEBJunc_Object_Condition/5(AEBJunc_PedTargetDXDY_observal) -> Bus Creator/3  "AEBJunc_PedTargetDXDY_observal"
  AEBJunc_Object_Condition/6(AEBJunc_PedTargetMovDir_observal) -> Bus Creator/4  "AEBJunc_PedTargetMovDir_observal"
  AEBJunc_Object_Condition/2(TOS_AEBJunc_VehTargets_Dx) -> AEBJuncTargetIndex/2(TOS_AEBJunc_ConditionPedTargets_Dx1)  "TOS_AEBJunc_VehTargets_Dx"
  AEBJunc_Object_Condition/7(AEBJunc_VehTargetFusionType_observal) -> Bus Creator/5  "AEBJunc_VehTargetFusionType_observal"
  AEBJunc_Object_Condition/8(AEBJunc_VehTargetObjectType_observal) -> Bus Creator/6  "AEBJunc_VehTargetObjectType_observal"
  AEBJunc_Object_Condition/9(AEBJunc_VehTargetDXDY_observal) -> Bus Creator/7  "AEBJunc_VehTargetDXDY_observal"
  AEBJunc_Object_Condition/10(AEBJunc_VehTargetMovDir_observal) -> Bus Creator/8  "AEBJunc_VehTargetMovDir_observal"
  Bus Selector3/14 -> AEBJunc_Object_Condition/14(Object_MovingState)  "<Object_MovingState>"
  AEBJunc_Object_Condition/11(AEBJunc_VehTargetMovState_observal) -> Bus Creator/9  "AEBJunc_VehTargetMovState_observal"
  Unit Delay3/1 -> AEBJunctionTargetInfor/5(AEBJunc_Target_ObjectType_K1)
  Subsystem1/2(ObjectType) -> Unit Delay3/1
  Unit Delay2/1 -> AEBJunctionTargetInfor/4(AEBJunc_Target_ObjectID_K1)
  [TOS_AEB_JAOBJ] -> Subsystem1/1(TOS_AEB_JAOBJ)
  Subsystem1/1(ObjectID) -> Unit Delay2/1
  From3/1 -> TOS_AEBLong_ObserVale/1(TOS_AEBJunc_TargetIndex)
  From4/1 -> TOS_AEBLong_ObserVale/2(TOS_AEBJunc_ObserVale)
  Bus Creator/1 -> [TOS_AEBJunc_ObserVale]  "TOS_AEBJunc_observal"
  AEBJunc_Object_Condition1/11(AEBJunc_VehTargetMovState_observal) -> Display10/1  "AEBJunc_VehTargetMovState_observal"
  Bus Selector1/14 -> Selector14/1  "<Object_MovingState>"
  AEBJunc_Object_Condition1/10(AEBJunc_VehTargetMovDir_observal) -> Display9/1  "AEBJunc_VehTargetMovDir_observal"
  AEBJunc_Object_Condition1/9(AEBJunc_VehTargetDXDY_observal) -> Display8/1  "AEBJunc_VehTargetDXDY_observal"
  AEBJunc_Object_Condition1/8(AEBJunc_VehTargetObjectType_observal) -> Display7/1  "AEBJunc_VehTargetObjectType_observal"
  AEBJunc_Object_Condition1/7(AEBJunc_VehTargetFusionType_observal) -> Display6/1  "AEBJunc_VehTargetFusionType_observal"
  AEBJunc_Object_Condition1/2(TOS_AEBJunc_VehTargets_Dx) -> Display1/1  "TOS_AEBJunc_VehTargets_Dx"
  AEBJunc_Object_Condition1/6(AEBJunc_PedTargetMovDir_observal) -> Display5/1  "AEBJunc_PedTargetMovDir_observal"
  AEBJunc_Object_Condition1/5(AEBJunc_PedTargetDXDY_observal) -> Display4/1  "AEBJunc_PedTargetDXDY_observal"
  AEBJunc_Object_Condition1/4(AEBJunc_PedTargetObjectType_observal) -> Display3/1  "AEBJunc_PedTargetObjectType_observal"
  Unit Delay5/1 -> AEBJunc_Object_Condition1/16(AEBJunc_Target_ObjectType_K1)
  Subsystem2/2(ObjectType) -> Unit Delay5/1
  AEBJunc_Object_Condition1/3(AEBJunc_PedTargetFusionType_observal) -> Display2/1  "AEBJunc_PedTargetFusionType_observal"
  Bus Selector1/13 -> AEBJunc_Object_Condition1/13(axvRefMs2)  "<axvRefMs2>"
  Bus Selector1/12 -> AEBJunc_Object_Condition1/12(psiDtOpt)  "<psiDtOpt>"
  Bus Selector1/3 -> Selector2/1  "<PP_ObjFusType_FR_Confirm>"
  Bus Selector1/11 -> AEBJunc_Object_Condition1/11(VIE_EgoVelocity)  "<vxvRefMs>"
  Bus Selector1/1 -> Selector10/1  "<Object_ID>"
  Bus Selector1/9 -> Selector8/1  "<Object_VX>"
  Unit Delay4/1 -> AEBJunc_Object_Condition1/15(AEBJunc_Target_ObjectID_K1)
  Bus Selector1/2 -> Selector1/1  "<PP_ObjFusType_FC_FR_Confirm>"
  Bus Selector1/8 -> Selector7/1  "<Object_HeadingAngle>"
  Bus Selector1/10 -> Selector9/1  "<Object_VY>"
  Bus Selector1/4 -> Selector3/1  "<Object_Type>"
  Bus Selector1/6 -> Selector5/1  "<Object_DY>"
  From2/1 -> Subsystem2/1(TOS_AEB_JAOBJ)
  Subsystem2/1(ObjectID) -> Unit Delay4/1
  Bus Selector1/7 -> Selector6/1  "<PP_ObjMovingDirSignalProcessing>"
  Bus Selector1/5 -> Selector4/1  "<Object_DX>"
  TOSAAt_OFM_TIL_VIE/1 -> Bus Selector2/1, Bus Selector3/1, Bus Selector1/1
  AEBJunc_Object_Condition1/1(TOS_AEBJunc_PedTargets_Dx) -> Display/1  "TOS_AEBJunc_ConditionPedTargets_Dx"
  Selector10/1 -> AEBJunc_Object_Condition1/1(Object_ID)
  Selector1/1 -> AEBJunc_Object_Condition1/2(PP_ObjFusType_FC_FR_Confirm)
  Selector2/1 -> AEBJunc_Object_Condition1/3(PP_ObjFusType_FR_Confirm)
  Selector3/1 -> AEBJunc_Object_Condition1/4(ObjectType)
  Selector4/1 -> AEBJunc_Object_Condition1/5(Object_Dx)
  Selector5/1 -> AEBJunc_Object_Condition1/6(Object_Dy)
  Selector6/1 -> AEBJunc_Object_Condition1/7(PP_ObjMovingDirSignalProcessing)
  Selector7/1 -> AEBJunc_Object_Condition1/8(Object_HeadingAngle)
  Selector8/1 -> AEBJunc_Object_Condition1/9(Object_VX)
  Selector9/1 -> AEBJunc_Object_Condition1/10(Object_VY)
  Selector14/1 -> AEBJunc_Object_Condition1/14(Object_MovingState)

== system PubIfDecisionTOS_MDL/TOS_20201112/TOS_2012080320/TOS/AEB/TOS_AEBJunct_20201208 ==
  TOSAAt_OFM_TIL_VIE : Inport
  AEBJuncTargetIndex : Subsystem
  AEBJunc_Object_Condition : Subsystem
  AEBJunc_Object_Condition1 : Subsystem  Commented=on
  AEBJunctionTargetInfor : Subsystem
  Bus Creator : BusCreator  Inputs=9
  Bus Selector1 : BusSelector  Commented=on  OutputSignals=OFM_SignalVerification.Object_ID,TOS_AddAttributes.PP_ObjFusType_FC_FR_Confirm,TOS_AddAttributes.PP_ObjFusType_FR_Confirm,OFM_SignalVerification.Object_Type,OFM_SignalVerification.Object_DX,OFM_SignalVerification.Object_DY,TOS_AddAttributes.PP_ObjMovingDirSignalProcessing,OFM_SignalVerification.Object_HeadingAngle,OFM_SignalVerification.Object_VX,OFM_SignalVerification.Object_VY,VIE_SignalVerification.vxvRefMs,VIE_SignalVerification.psiDtOpt,VIE_SignalVerification.axvRefMs2,OFM_SignalVerification.Object_MovingState
  Bus Selector2 : BusSelector  OutputSignals=OFM_SignalVerification,TOS_AddAttributes
  Bus Selector3 : BusSelector  OutputSignals=OFM_SignalVerification.Object_ID,TOS_AddAttributes.PP_ObjFusType_FC_FR_Confirm,TOS_AddAttributes.PP_ObjFusType_FR_Confirm,OFM_SignalVerification.Object_Type,OFM_SignalVerification.Object_DX,OFM_SignalVerification.Object_DY,TOS_AddAttributes.PP_ObjMovingDirSignalProcessing,OFM_SignalVerification.Object_HeadingAngle,OFM_SignalVerification.Object_VX,OFM_SignalVerification.Object_VY,VIE_SignalVerification.vxvRefMs,VIE_SignalVerification.psiDtOpt,VIE_SignalVerification.axvRefMs2,OFM_SignalVerification.Object_MovingState
  Display{,1..10} (11 alike) : Display  Commented=on
  From2 : From  Commented=on  GotoTag=TOS_AEB_JAOBJ
  From3 : From  Commented=on  GotoTag=TOS_AEBJunc_TargetIndex
  From4 : From  Commented=on  GotoTag=TOS_AEBJunc_ObserVale
  Selector{1..10,14} (11 alike) : Selector  Commented=on  InputPortWidth=80  IndexOptions=Index vector (dialog)  Indices=60  OutputSizes=1
  Subsystem : Subsystem
  Subsystem1 : Subsystem
  Subsystem2 : Subsystem  Commented=on
  TOS_AEBLong_ObserVale : Subsystem  Commented=on
  Unit Delay{,1..3} (4 alike) : UnitDelay  SampleTime=-1  HasFrameUpgradeWarning=on
  Unit Delay4 : UnitDelay  Commented=on  SampleTime=-1  HasFrameUpgradeWarning=on
  Unit Delay5 : UnitDelay  Commented=on  SampleTime=-1  HasFrameUpgradeWarning=on
  TOS_AEB_JAOBJ : Outport
  wires:
  AEBJuncTargetIndex/1(TOS_AEBJuncTargetIndex) -> [TOS_AEBJunc_TargetIndex], AEBJunctionTargetInfor/3(TOS_AEBJuncTargetIndex)  "TOS_AEBJunc_Index"
  AEBJunc_Object_Condition/1(TOS_AEBJunc_PedTargets_Dx) -> AEBJuncTargetIndex/1(TOS_AEBJunc_ConditionPedTargets_Dx)  "TOS_AEBJunc_ConditionPedTargets_Dx"
  AEBJunctionTargetInfor/1(TOS_AEB_JAOBJ) -> [TOS_AEB_JAOBJ], TOS_AEB_JAOBJ/1
  Bus Selector2/1 -> AEBJunctionTargetInfor/1(OFM_SignalVerification)  "<OFM_SignalVerification>"
  Bus Selector2/2 -> AEBJunctionTargetInfor/2(TOS_AddAttributes)  "<TOS_AddAttributes>"
  Bus Selector3/5 -> AEBJunc_Object_Condition/5(Object_Dx)  "<Object_DX>"
  Bus Selector3/7 -> AEBJunc_Object_Condition/7(PP_ObjMovingDirSignalProcessing)  "<PP_ObjMovingDirSignalProcessing>"
  Subsystem/1(ObjectID) -> Unit Delay/1
  [TOS_AEB_JAOBJ] -> Subsystem/1(TOS_AEB_JAOBJ)
  Bus Selector3/6 -> AEBJunc_Object_Condition/6(Object_Dy)  "<Object_DY>"
  Bus Selector3/4 -> AEBJunc_Object_Condition/4(ObjectType)  "<Object_Type>"
  Bus Selector3/10 -> AEBJunc_Object_Condition/10(Object_VY)  "<Object_VY>"
  Bus Selector3/8 -> AEBJunc_Object_Condition/8(Object_HeadingAngle)  "<Object_HeadingAngle>"
  Bus Selector3/2 -> AEBJunc_Object_Condition/2(PP_ObjFusType_FC_FR_Confirm)  "<PP_ObjFusType_FC_FR_Confirm>"
  Unit Delay/1 -> AEBJunc_Object_Condition/15(AEBJunc_Target_ObjectID_K1)
  Bus Selector3/9 -> AEBJunc_Object_Condition/9(Object_VX)  "<Object_VX>"
  Bus Selector3/1 -> AEBJunc_Object_Condition/1(Object_ID)  "<Object_ID>"
  Bus Selector3/11 -> AEBJunc_Object_Condition/11(VIE_EgoVelocity)  "<vxvRefMs>"
  Bus Selector3/3 -> AEBJunc_Object_Condition/3(PP_ObjFusType_FR_Confirm)  "<PP_ObjFusType_FR_Confirm>"
  Bus Selector3/12 -> AEBJunc_Object_Condition/12(psiDtOpt)  "<psiDtOpt>"
  Bus Selector3/13 -> AEBJunc_Object_Condition/13(axvRefMs2)  "<axvRefMs2>"
  AEBJunc_Object_Condition/3(AEBJunc_PedTargetFusionType_observal) -> Bus Creator/1  "TOS_AEBJunc_PedTargetFusionType_observal"
  Subsystem/2(ObjectType) -> Unit Delay1/1
  Unit Delay1/1 -> AEBJunc_Object_Condition/16(AEBJunc_Target_ObjectType_K1)
  AEBJunc_Object_Condition/4(AEBJunc_PedTargetObjectType_observal) -> Bus Creator/2  "TOS_AEBJunc_PedTargetObjectType_observal"
  AEBJunc_Object_Condition/5(AEBJunc_PedTargetDXDY_observal) -> Bus Creator/3  "TOS_AEBJunc_PedTargetDXDY_observal"
  AEBJunc_Object_Condition/6(AEBJunc_PedTargetMovDir_observal) -> Bus Creator/4  "TOS_AEBJunc_PedTargetMovDir_observal"
  AEBJunc_Object_Condition/2(TOS_AEBJunc_VehTargets_Dx) -> AEBJuncTargetIndex/2(TOS_AEBJunc_ConditionPedTargets_Dx1)  "TOS_AEBJunc_VehTargets_Dx"
  AEBJunc_Object_Condition/7(AEBJunc_VehTargetFusionType_observal) -> Bus Creator/5  "TOS_AEBJunc_VehTargetFusionType_observal"
  AEBJunc_Object_Condition/8(AEBJunc_VehTargetObjectType_observal) -> Bus Creator/6  "TOS_AEBJunc_VehTargetObjectType_observal"
  AEBJunc_Object_Condition/9(AEBJunc_VehTargetDXDY_observal) -> Bus Creator/7  "TOS_AEBJunc_VehTargetDXDY_observal"
  AEBJunc_Object_Condition/10(AEBJunc_VehTargetMovDir_observal) -> Bus Creator/8  "TOS_AEBJunc_VehTargetMovDir_observal"
  Bus Selector3/14 -> AEBJunc_Object_Condition/14(Object_MovingState)  "<Object_MovingState>"
  AEBJunc_Object_Condition/11(AEBJunc_VehTargetMovState_observal) -> Bus Creator/9  "TOS_AEBJunc_VehTargetMovState_observal"
  Unit Delay3/1 -> AEBJunctionTargetInfor/5(AEBJunc_Target_ObjectType_K1)
  Subsystem1/2(ObjectType) -> Unit Delay3/1
  Unit Delay2/1 -> AEBJunctionTargetInfor/4(AEBJunc_Target_ObjectID_K1)
  [TOS_AEB_JAOBJ] -> Subsystem1/1(TOS_AEB_JAOBJ)
  Subsystem1/1(ObjectID) -> Unit Delay2/1
  From3/1 -> TOS_AEBLong_ObserVale/1(TOS_AEBJunc_TargetIndex)
  From4/1 -> TOS_AEBLong_ObserVale/2(TOS_AEBJunc_ObserVale)
  Bus Creator/1 -> [TOS_AEBJunc_ObserVale]  "TOS_AEBJunc_observal"
  AEBJunc_Object_Condition1/11(AEBJunc_VehTargetMovState_observal) -> Display10/1  "AEBJunc_VehTargetMovState_observal"
  Bus Selector1/14 -> Selector14/1  "<Object_MovingState>"
  AEBJunc_Object_Condition1/10(AEBJunc_VehTargetMovDir_observal) -> Display9/1  "AEBJunc_VehTargetMovDir_observal"
  AEBJunc_Object_Condition1/9(AEBJunc_VehTargetDXDY_observal) -> Display8/1  "AEBJunc_VehTargetDXDY_observal"
  AEBJunc_Object_Condition1/8(AEBJunc_VehTargetObjectType_observal) -> Display7/1  "AEBJunc_VehTargetObjectType_observal"
  AEBJunc_Object_Condition1/7(AEBJunc_VehTargetFusionType_observal) -> Display6/1  "AEBJunc_VehTargetFusionType_observal"
  AEBJunc_Object_Condition1/2(TOS_AEBJunc_VehTargets_Dx) -> Display1/1  "TOS_AEBJunc_VehTargets_Dx"
  AEBJunc_Object_Condition1/6(AEBJunc_PedTargetMovDir_observal) -> Display5/1  "AEBJunc_PedTargetMovDir_observal"
  AEBJunc_Object_Condition1/5(AEBJunc_PedTargetDXDY_observal) -> Display4/1  "AEBJunc_PedTargetDXDY_observal"
  AEBJunc_Object_Condition1/4(AEBJunc_PedTargetObjectType_observal) -> Display3/1  "AEBJunc_PedTargetObjectType_observal"
  Unit Delay5/1 -> AEBJunc_Object_Condition1/16(AEBJunc_Target_ObjectType_K1)
  Subsystem2/2(ObjectType) -> Unit Delay5/1
  AEBJunc_Object_Condition1/3(AEBJunc_PedTargetFusionType_observal) -> Display2/1  "AEBJunc_PedTargetFusionType_observal"
  Bus Selector1/13 -> AEBJunc_Object_Condition1/13(axvRefMs2)  "<axvRefMs2>"
  Bus Selector1/12 -> AEBJunc_Object_Condition1/12(psiDtOpt)  "<psiDtOpt>"
  Bus Selector1/3 -> Selector2/1  "<PP_ObjFusType_FR_Confirm>"
  Bus Selector1/11 -> AEBJunc_Object_Condition1/11(VIE_EgoVelocity)  "<vxvRefMs>"
  Bus Selector1/1 -> Selector10/1  "<Object_ID>"
  Bus Selector1/9 -> Selector8/1  "<Object_VX>"
  Unit Delay4/1 -> AEBJunc_Object_Condition1/15(AEBJunc_Target_ObjectID_K1)
  Bus Selector1/2 -> Selector1/1  "<PP_ObjFusType_FC_FR_Confirm>"
  Bus Selector1/8 -> Selector7/1  "<Object_HeadingAngle>"
  Bus Selector1/10 -> Selector9/1  "<Object_VY>"
  Bus Selector1/4 -> Selector3/1  "<Object_Type>"
  Bus Selector1/6 -> Selector5/1  "<Object_DY>"
  From2/1 -> Subsystem2/1(TOS_AEB_JAOBJ)
  Subsystem2/1(ObjectID) -> Unit Delay4/1
  Bus Selector1/7 -> Selector6/1  "<PP_ObjMovingDirSignalProcessing>"
  Bus Selector1/5 -> Selector4/1  "<Object_DX>"
  TOSAAt_OFM_TIL_VIE/1 -> Bus Selector2/1, Bus Selector3/1, Bus Selector1/1
  AEBJunc_Object_Condition1/1(TOS_AEBJunc_PedTargets_Dx) -> Display/1  "TOS_AEBJunc_ConditionPedTargets_Dx"
  Selector10/1 -> AEBJunc_Object_Condition1/1(Object_ID)
  Selector1/1 -> AEBJunc_Object_Condition1/2(PP_ObjFusType_FC_FR_Confirm)
  Selector2/1 -> AEBJunc_Object_Condition1/3(PP_ObjFusType_FR_Confirm)
  Selector3/1 -> AEBJunc_Object_Condition1/4(ObjectType)
  Selector4/1 -> AEBJunc_Object_Condition1/5(Object_Dx)
  Selector5/1 -> AEBJunc_Object_Condition1/6(Object_Dy)
  Selector6/1 -> AEBJunc_Object_Condition1/7(PP_ObjMovingDirSignalProcessing)
  Selector7/1 -> AEBJunc_Object_Condition1/8(Object_HeadingAngle)
  Selector8/1 -> AEBJunc_Object_Condition1/9(Object_VX)
  Selector9/1 -> AEBJunc_Object_Condition1/10(Object_VY)
  Selector14/1 -> AEBJunc_Object_Condition1/14(Object_MovingState)

== system PubIfDecisionTOS_MDL/TOS_20201112/TOS_2012080320/TOS/AEB/TOS_AEBLatCro1105 ==
  TOSAAt_OFM_TIL_VIE : Inport
  AEBLatTrgInfor : Subsystem
  AEBLat_Object_Condition : Subsystem
  AEBLat_Object_Condition2 : Subsystem  Commented=on
  AEBLat_TargetIndex : Subsystem
  Bus Creator : BusCreator  Inputs=4
  Bus Selector1 : BusSelector  OutputSignals=OFM_SignalVerification.Object_ID,TOS_AddAttributes.PP_ObjFusType_FC_FR_Confirm,TOS_AddAttributes.PP_ObjFusType_FR_Confirm,OFM_SignalVerification.Object_Type,OFM_SignalVerification.Object_DX,OFM_SignalVerification.Object_DY,TOS_AddAttributes.PP_ObjMovingDirSignalProcessing,OFM_SignalVerification.Object_HeadingAngle,OFM_SignalVerification.Object_VX,OFM_SignalVerification.Object_VY,VIE_SignalVerification.vxvRefMs,VIE_SignalVerification.psiDtOpt
  Bus Selector2 : BusSelector  OutputSignals=OFM_SignalVerification,TOS_AddAttributes
  Bus Selector4 : BusSelector  Commented=on  OutputSignals=OFM_SignalVerification.Object_ID,TOS_AddAttributes.PP_ObjFusType_FC_FR_Confirm,TOS_AddAttributes.PP_ObjFusType_FR_Confirm,OFM_SignalVerification.Object_Type,OFM_SignalVerification.Object_DX,OFM_SignalVerification.Object_DY,TOS_AddAttributes.PP_ObjMovingDirSignalProcessing,OFM_SignalVerification.Object_HeadingAngle,OFM_SignalVerification.Object_VX,OFM_SignalVerification.Object_VY,VIE_SignalVerification.vxvRefMs,VIE_SignalVerification.psiDtOpt
  Display{5..9} (5 alike) : Display  Commented=on
  From2 : From  Commented=on  GotoTag=TOS_AEB_LATOBJ
  Selector{10..19} (10 alike) : Selector  Commented=on  InputPortWidth=80  IndexOptions=Index vector (dialog)  Indices=64  OutputSizes=1
  Subsystem : Subsystem
  Subsystem1 : Subsystem
  Subsystem2 : Subsystem  Commented=on
  Terminator : Terminator
  Unit Delay{,1,3..4} (4 alike) : UnitDelay  SampleTime=-1  HasFrameUpgradeWarning=on
  Unit Delay2 : UnitDelay  Commented=on  SampleTime=-1  HasFrameUpgradeWarning=on
  TOS_AEB_LATOBJ : Outport
  wires:
  Bus Selector1/3 -> AEBLat_Object_Condition/3(PP_ObjFusType_FR_Confirm)  "<PP_ObjFusType_FR_Confirm>"
  Bus Selector1/2 -> AEBLat_Object_Condition/2(PP_ObjFusType_FC_FR_Confirm)  "<PP_ObjFusType_FC_FR_Confirm>"
  Bus Selector1/11 -> AEBLat_Object_Condition/11(VIE_EgoVelocity)  "<vxvRefMs>"
  Bus Selector1/10 -> AEBLat_Object_Condition/10(Object_VY)  "<Object_VY>"
  Bus Selector1/9 -> AEBLat_Object_Condition/9(Object_VX)  "<Object_VX>"
  Bus Selector1/8 -> AEBLat_Object_Condition/8(Object_HeadingAngle)  "<Object_HeadingAngle>"
  Bus Selector1/7 -> AEBLat_Object_Condition/7(PP_ObjMovingDirSignalProcessing)  "<PP_ObjMovingDirSignalProcessing>"
  Bus Selector1/1 -> AEBLat_Object_Condition/1(Object_ID)  "<Object_ID>"
  Bus Selector1/4 -> AEBLat_Object_Condition/4(ObjectType)  "<Object_Type>"
  Bus Selector2/1 -> AEBLatTrgInfor/1(OFM_SignalVerification)  "<OFM_SignalVerification>"
  Bus Selector2/2 -> AEBLatTrgInfor/2(TOS_AddAttributes)  "<TOS_AddAttributes>"
  Bus Selector1/5 -> AEBLat_Object_Condition/5(Object_Dx)  "<Object_DX>"
  Bus Selector1/6 -> AEBLat_Object_Condition/6(Object_Dy)  "<Object_DY>"
  AEBLat_TargetIndex/1(AEBLat_Target_Index) -> AEBLatTrgInfor/3(TOS_AEBLatTrg_Index)  "TOS_AEBLat_Index"
  AEBLat_Object_Condition/1(TOS_AEBLat_ConditionTargets_Dx) -> AEBLat_TargetIndex/1(TOS_AEBLat_Targets_Dx)  "TOS_AEBLat_ConditionTargets_Dx"
  AEBLat_Object_Condition/2(AEBLat_TargetFusionType_observal) -> Bus Creator/1  "AEBLat_TargetFusionType_observal"
  AEBLat_Object_Condition/3(AEBLat_TargetObjectType_observal) -> Bus Creator/2  "AEBLat_TargetObjectType_observal"
  AEBLat_Object_Condition/4(AEBLat_TargetDXDY_observal) -> Bus Creator/3  "AEBLat_TargetDXDY_observal"
  AEBLat_Object_Condition/5(AEBLat_TargetMovDir_observal) -> Bus Creator/4  "AEBLat_TargetMovDir_observal"
  AEBLatTrgInfor/1(TOS_AEB_LATOBJ) -> [TOS_AEB_LATOBJ], TOS_AEB_LATOBJ/1
  Bus Selector1/12 -> AEBLat_Object_Condition/12(psiDtOpt)  "<psiDtOpt>"
  [TOS_AEB_LATOBJ] -> Subsystem/1(TOS_AEB_LATOBJ)
  Subsystem/1(ObjectID) -> Unit Delay/1
  Unit Delay/1 -> AEBLat_Object_Condition/13(AEBLat_Target_ObjectID_K1)
  Selector18/1 -> AEBLat_Object_Condition2/9(Object_VX)
  Selector19/1 -> AEBLat_Object_Condition2/10(Object_VY)
  Selector16/1 -> AEBLat_Object_Condition2/7(PP_ObjMovingDirSignalProcessing)
  Selector17/1 -> AEBLat_Object_Condition2/8(Object_HeadingAngle)
  Selector15/1 -> AEBLat_Object_Condition2/6(Object_Dy)
  Selector14/1 -> AEBLat_Object_Condition2/5(Object_Dx)
  Selector13/1 -> AEBLat_Object_Condition2/4(ObjectType)
  Selector12/1 -> AEBLat_Object_Condition2/3(PP_ObjFusType_FR_Confirm)
  Selector11/1 -> AEBLat_Object_Condition2/2(PP_ObjFusType_FC_FR_Confirm)
  Selector10/1 -> AEBLat_Object_Condition2/1(Object_ID)
  Bus Selector4/3 -> Selector12/1  "<PP_ObjFusType_FR_Confirm>"
  Bus Selector4/2 -> Selector11/1  "<PP_ObjFusType_FC_FR_Confirm>"
  Bus Selector4/11 -> AEBLat_Object_Condition2/11(VIE_EgoVelocity)  "<vxvRefMs>"
  Bus Selector4/10 -> Selector19/1  "<Object_VY>"
  Bus Selector4/9 -> Selector18/1  "<Object_VX>"
  Bus Selector4/8 -> Selector17/1  "<Object_HeadingAngle>"
  Bus Selector4/7 -> Selector16/1  "<PP_ObjMovingDirSignalProcessing>"
  Bus Selector4/1 -> Selector10/1  "<Object_ID>"
  Bus Selector4/4 -> Selector13/1  "<Object_Type>"
  Bus Selector4/5 -> Selector14/1  "<Object_DX>"
  Bus Selector4/6 -> Selector15/1  "<Object_DY>"
  TOSAAt_OFM_TIL_VIE/1 -> Bus Selector2/1, Bus Selector4/1, Bus Selector1/1
  Bus Selector4/12 -> AEBLat_Object_Condition2/12(psiDtOpt)  "<psiDtOpt>"
  From2/1 -> Subsystem2/1(TOS_AEB_LATOBJ)
  Subsystem2/1(ObjectID) -> Unit Delay2/1
  Unit Delay2/1 -> AEBLat_Object_Condition2/13(AEBLat_Target_ObjectID_K1)
  AEBLat_Object_Condition2/5(AEBLat_TargetMovDir_observal) -> Display9/1
  AEBLat_Object_Condition2/4(AEBLat_TargetDXDY_observal) -> Display8/1
  AEBLat_Object_Condition2/3(AEBLat_TargetObjectType_observal) -> Display7/1
  AEBLat_Object_Condition2/2(AEBLat_TargetFusionType_observal) -> Display6/1
  AEBLat_Object_Condition2/1(TOS_AEBLat_ConditionTargets_Dx) -> Display5/1
  Subsystem/2(ObjectType) -> Unit Delay3/1
  Unit Delay3/1 -> AEBLat_Object_Condition/14(AEBLat_Target_ObjectType_K1)
  Unit Delay4/1 -> AEBLatTrgInfor/5(AEBLat_Target_ObjectType_K1)
  Subsystem1/2(ObjectType) -> Unit Delay4/1
  Unit Delay1/1 -> AEBLatTrgInfor/4(AEBLat_Target_ObjectID_K1)
  Subsystem1/1(ObjectID) -> Unit Delay1/1
  [TOS_AEB_LATOBJ] -> Subsystem1/1(TOS_AEB_LATOBJ)
  Bus Creator/1 -> Terminator/1  "TOS_AEBLat_ObserVal"
